simulink model "addition"  (R2020b)
settings: Solver=VariableStepAuto  StartTime=0.0  StopTime=10.0  RelTol=1e-3
settings Model: Creator=tsmith  LastModifiedBy=tsmith

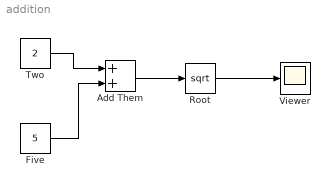
== system addition ==
  Add Them : Sum
  Five : Constant  Value=5
  Root : Sqrt  SaturateOnIntegerOverflow=on
  Two : Constant  Value=2
  Viewer : Scope
  wires:
  Two/1 -> Add Them/1
  Five/1 -> Add Them/2
  Add Them/1 -> Root/1
  Root/1 -> Viewer/1
